simulink model "step1"  (R2018b)
settings: Solver=ode3  StartTime=0.0  StopTime=inf  RelTol=1e-3  EnableMultiTasking=on
libraries: legoev3lib x4
settings Model: FPTRunName=Active  ExtModeTrigDuration=2  Creator=tom  LastModifiedBy=tom
settings SolverCC: PositivePriorityOrder=on
settings DataIOCC: LimitDataPoints=on  SaveFormat=Array
settings OptimizationCC: ExpressionDepthLimit=2147483647  LifeSpan=Inf  MaxStackSize=64
settings DebuggingCC: UnderspecifiedInitializationDetection=Classic  MergeDetectMultiDrivingBlocksExec=none  FcnCallInpInsideContextMsg=warning  AllowSymbolicDim=off  StateNameClashWarn=warning  SFUnexpectedBacktrackingDiag=warning  SFNoUnconditionalDefaultTransitionDiag=warning  SFExecutionAtInitializationDiag=none
settings HardwareCC: ProdBitPerPointer=32  ProdBitPerSizeT=32  ProdBitPerPtrDiffT=32  ProdLargestAtomicInteger=Long  ProdWordSize=32  ProdHWDeviceType=ARM Compatible->ARM 9  UseEmbeddedCoderFeatures=off  UseSimulinkCoderFeatures=off
settings ModelReferenceCC: PropagateSignalLabelsOutOfModel=off
settings SFSimCC: SimUseLocalCustomCode=off
settings RTWCC: SystemTargetFile=ert.tlc  HardwareBoard=LEGO MINDSTORMS EV3  TemplateMakefile=ert_default_tmf  GenerateReport=on  RTWVerbose=off  RTWUseLocalCustomCode=off  Toolchain=Sourcery G++ Lite v2009q3  BuildConfiguration=Faster Runs  LaunchReport=on
settings CodeAppCC: ForceParamTrailComments=on  OperatorAnnotations=on  StateflowObjectComments=on  MATLABSourceComments=on
settings ERTTargetCC: MultiwordLength=2048  ERTCustomFileBanners=off  SupportContinuousTime=on  SupportNonInlinedSFcns=on  RemoveResetFunc=off  SupportVariableSizeSignals=on  ModelStepFunctionPrototypeControlCompliant=off
settings ConfigComp: CovMetricSettings=dw  CovHtmlReporting=on  CovSaveCumulativeToWorkspaceVar=on  CovSaveSingleToWorkspaceVar=on  CovExternalEMLEnable=off  CovSFcnEnable=off

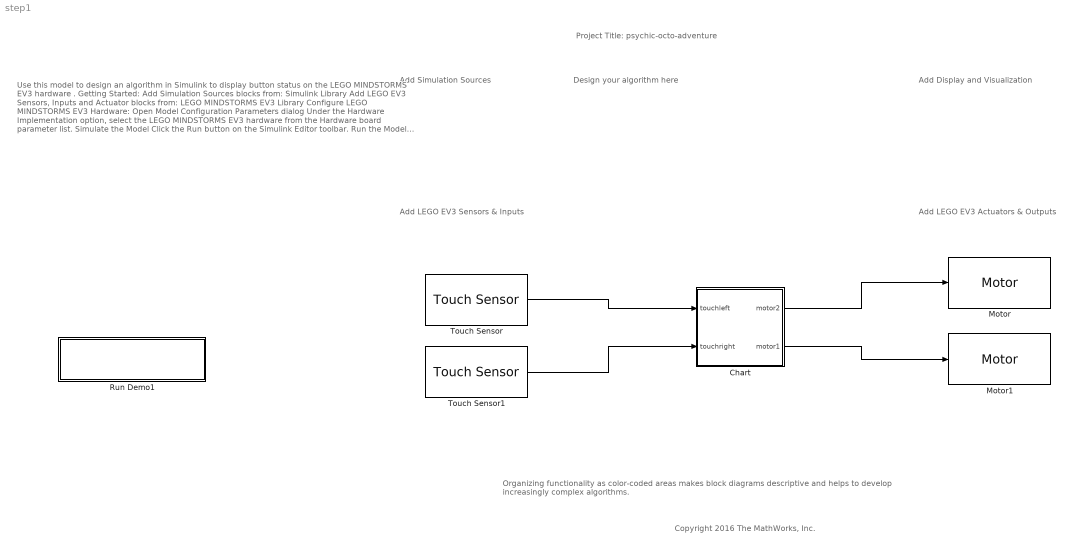
== system step1 ==
  note: Project Title: psychic-octo-adventure
  note: Copyright 2016 The MathWorks, Inc.
  note: Add LEGO EV3 Sensors & Inputs
  note: Add LEGO EV3 Actuators & Outputs
  note: Add Display and Visualization
  note: Design your algorithm here
  note: Add Simulation Sources
  note: Use this model to design an algorithm in Simulink to display button status on the LEGO MINDSTORMS EV3 hardware .
      |
      | Getting Started:
      |
      | Add Simulation Sources blocks from:
      | Simulink Library
      | Add LEGO EV3 Sensors, Inputs and Actuator blocks from:
      | LEGO MINDSTORMS EV3 Library
      |
      | Configure LEGO MINDSTORMS EV3 Hardware:
      |
      | Open Model Configuration Parameters dialog
      | Under the Hardware Implementation option, select the LEGO MINDSTORMS EV3 hardware from the Hardware board parameter list.
      |
      | Simulate the Model
      |
      | Click the Run button on the Simulink Editor toolbar.
      |
      | Run the Model on LEGO MINDSTORMS EV3 Hardware
      |
      | Click the Deploy to Hardware button on the Simulink Editor toolbar.
      |
      | Other Things to Try:
      |
      | Create and run a model that detects the obstacle and stops the LEGO EV3 robot. HINT: Use Ultrasonic Sensor and Motor blocks.
  note: Organizing functionality as color-coded areas makes block diagrams descriptive and helps to develop increasingly complex algorithms.
  Chart : Stateflow chart  TreatAsAtomicUnit=on
  Motor : legoev3lib/Motor  sportNumber=B  sstopAction=Brake
  Motor1 : legoev3lib/Motor  sportNumber=C  sstopAction=Brake
  Run Demo1 : Subsystem  Description=Controls host-side RTDX processing.
      mask Display: pic=imread('ev3DeploytoHardware.png');image(pic);
  Touch Sensor : legoev3lib/Touch Sensor  portNumber=1  sampleTime=0.1
      settings: SourceProductName=Simulink Support Package for LEGO MINDSTORMS EV3 Hardware  SourceProductBaseCode=LEGOEV3
  Touch Sensor1 : legoev3lib/Touch Sensor  portNumber=2  sampleTime=0.1
      settings: SourceProductName=Simulink Support Package for LEGO MINDSTORMS EV3 Hardware  SourceProductBaseCode=LEGOEV3
  wires:
  Chart/1(motor2) -> Motor/1
  Chart/2(motor1) -> Motor1/1
  Touch Sensor/1 -> Chart/1(touchleft)
  Touch Sensor1/1 -> Chart/2(touchright)

== system step1/Run Demo1 ==

== stateflow chart step1/Chart ==
  state RESET
  state TURNLEFT
    entry:
    motor1 = 23
    motor2 = -23
  state MANUAL
    entry:
    motor1 = 0;
    motor2 = 0;
  state AUTONOMOUS1
    entry:
    motor1 = 100
    motor2 = -100
  state HOLD
  state STOP
  state FORWARD
    entry:
    motor1 = 30;
    motor2 = 30;
  state TURNRIGHT
    entry:
    motor1 = -23
    motor2 = 23
  RESET -> MANUAL [order 1] : after(1, sec)
  AUTONOMOUS1 -> RESET : [touchleft == 1 & touchright == 1]
  RESET -> AUTONOMOUS1 [order 2] : [not(touchleft == 1 & touchright == 1)]
  (default) -> MANUAL
  TURNLEFT -> MANUAL : [not(touchleft == 1 & touchright == 0)]
  MANUAL -> TURNLEFT [order 1] : [touchleft == 1 & touchright == 0]
  MANUAL -> HOLD [order 3] : [touchleft == 1 & touchright == 1]
  HOLD -> AUTONOMOUS1 [order 2] : after(1, sec)
  HOLD -> FORWARD [order 1] : [not(touchleft == 1 & touchright == 1)]
  STOP -> MANUAL : [touchleft == 0 & touchright == 0]
  FORWARD -> STOP : [not(touchleft == 0 & touchright == 0)]
  TURNRIGHT -> MANUAL : [not(touchleft == 0 & touchright == 1)]
  MANUAL -> TURNRIGHT [order 2] : [touchleft == 0 & touchright == 1]
  data: touchleft input; motor2 output; motor1 output; touchright input
